simulink model "Project_v1"  (R2022a)
settings: Solver=VariableStepAuto  StartTime=0.0  StopTime=10.0  RelTol=1e-3
libraries: simulink x4
settings Model: Creator=AAMIR  LastModifiedBy=AAMIR

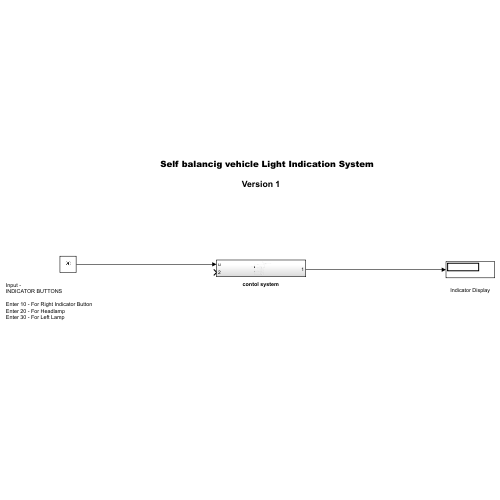
[thumbnail: Simulink's stored preview of the top-level diagram]
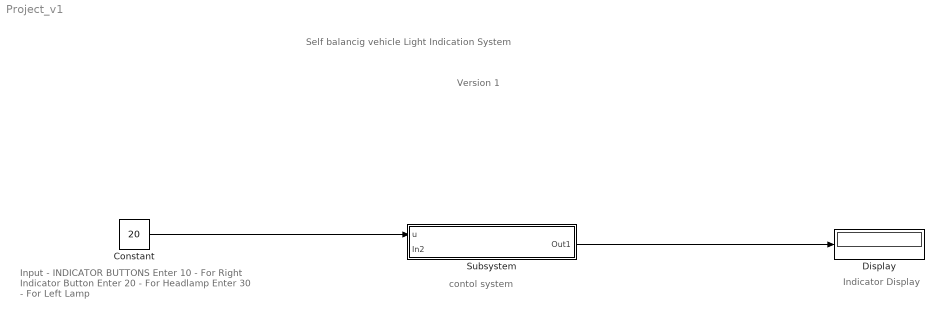
== system Project_v1 ==
  note: Version 1
  note: Self balancig vehicle Light Indication System
  note: contol system
  note: Input -
      | INDICATOR BUTTONS
      |
      | Enter 10 - For Right Indicator Button
      | Enter 20 - For Headlamp
      | Enter 30 - For Left Lamp
  note: Indicator Display
  Constant : Constant  Value=20
  Display : Display
  Subsystem : Subsystem
  wires:
  Constant/1 -> Subsystem/1(u)
  Subsystem/1(Out1) -> Display/1

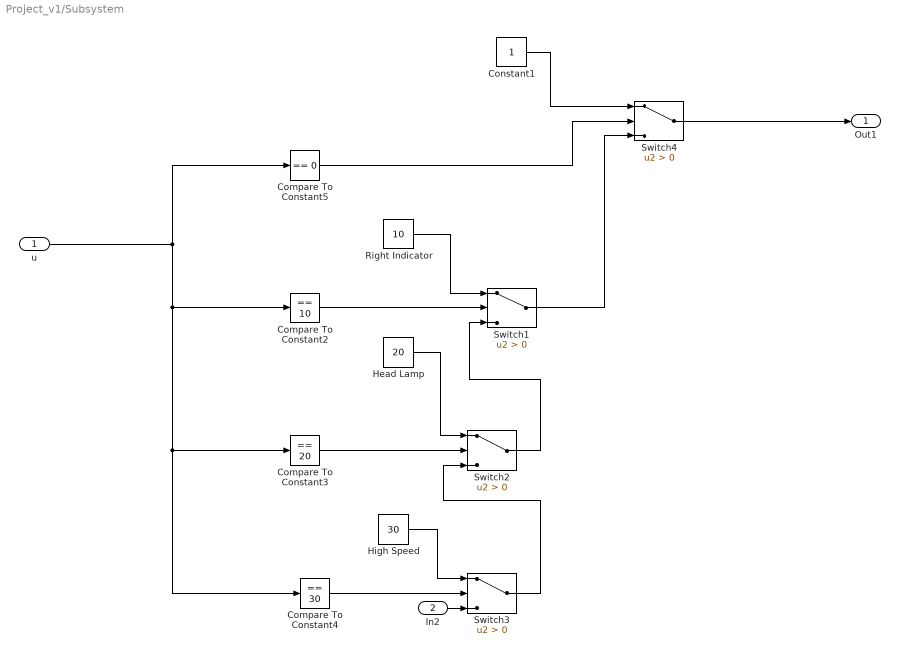
== system Project_v1/Subsystem ==
  u : Inport
  In2 : Inport  Port=2
  Compare To Constant2 : simulink/Logic and Bit Operations/Compare To Constant  relop===  const=10  OutDataTypeStr=boolean
  Compare To Constant3 : simulink/Logic and Bit Operations/Compare To Constant  relop===  const=20  OutDataTypeStr=boolean
  Compare To Constant4 : simulink/Logic and Bit Operations/Compare To Constant  relop===  const=30  OutDataTypeStr=boolean
  Compare To Constant5 : simulink/Logic and Bit Operations/Compare To Constant  relop===  const=0  OutDataTypeStr=boolean
  Constant1 : Constant
  Head Lamp : Constant  Value=20
  High Speed : Constant  Value=30
  Right Indicator : Constant  Value=10
  Switch{1..4} (4 alike) : Switch  Criteria=u2 > Threshold  SaturateOnIntegerOverflow=off  InputSameDT=off
  Out1 : Outport
  wires:
  Compare To Constant2/1 -> Switch1/2
  Switch2/1 -> Switch1/3
  u/1 -> Compare To Constant4/1, Compare To Constant3/1, Compare To Constant2/1, Compare To Constant5/1
  Switch1/1 -> Switch4/3
  Compare To Constant5/1 -> Switch4/2
  Head Lamp/1 -> Switch2/1
  Compare To Constant4/1 -> Switch3/2
  Switch3/1 -> Switch2/3
  Right Indicator/1 -> Switch1/1
  High Speed/1 -> Switch3/1
  Compare To Constant3/1 -> Switch2/2
  Constant1/1 -> Switch4/1
  Switch4/1 -> Out1/1
  In2/1 -> Switch3/3
